simulink model "vkr_ch2_sync_custom"  (R2025b)
settings: Solver=FixedStepDiscrete  StartTime=0.0  StopTime=Nsym/Rs  FixedStep=1/Fs_tx  RelTol=1e-3
values from neighbouring files (symbols this model uses):
  Fs_tx = Rs * sps_tx    (= 8000000)    [params_tx.m]    (also in test_sync_loop.m)
  k_bits = log2(M)    [compare_all_architectures.m]    (also in compare_round_period_ber.m; compare_sync_direct.m; params_tx.m; run_ber_curve.m)
  Nsym = 10000    [params_tx.m]    (also in run_dynamics.m = 2000; run_sco_test.m = 30000; test_modelsim_io.m = 5000; test_rice_loop.m = 5000)
  rolloff = 0.35    [compare_all_architectures.m]    (also in compare_round_period_ber.m; compare_sync_direct.m; params_tx.m; process_real_data.m = 0.2)
  Rs = 1e6    (= 1000000)    [params_tx.m]    (also in test_sync_loop.m)
  sps_tx = 40    [compare_all_architectures.m]    (also in compare_round_period_ber.m; compare_sync_direct.m = 8; params_tx.m = 8; run_ber_curve.m = 8)
  timing_offset = 0.3    [compare_all_architectures.m]    (also in compare_round_period_ber.m; compare_sync_direct.m; params_tx.m; run_ber_curve.m)
libraries: commfilt2 x2, commchan3 x1, commrandsrc3 x1, commdigbbndpm3 x1, commsync2 x1, dspsigops x1
settings Model: Creator=Gostie2k  LastModifiedBy=t-kudimov

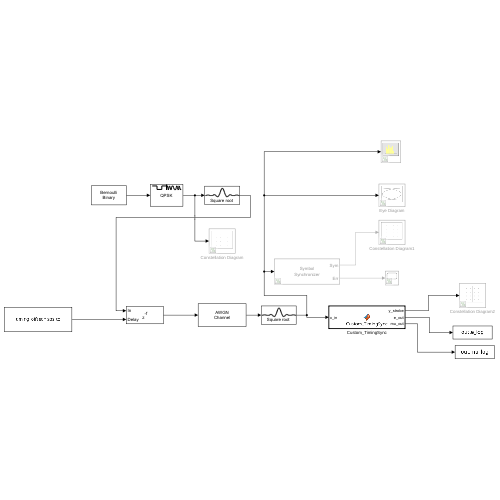
[thumbnail: Simulink's stored preview of the top-level diagram]
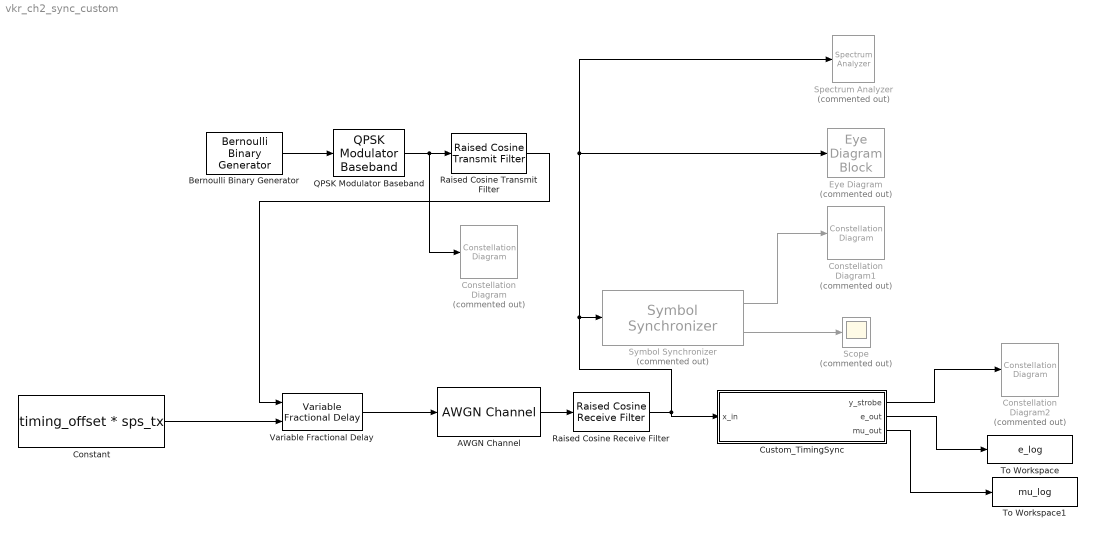
== system vkr_ch2_sync_custom ==
  AWGN Channel : commchan3/AWGN Channel  LegacyMode=off  NoiseMethod="Signal to noise ratio  (Eb/No)"  noiseMode="Signal to noise ratio  (SNR)"  EbNo=EbNo_dB  EsNo=10  SNR=10  BitsPerSymbol=k_bits  SignalPower=1  SpecifySymbolPeriod=off  SamplesPerSymbol=sps_tx  SymbolPeriod=1  VarianceSource=Parameter  Variance=1  RandomStream=Global stream  Seed=67  SimulateUsing=Code generation
  Bernoulli Binary Generator : commrandsrc3/Bernoulli Binary Generator  ProbabilityOfZero=0.5  SeedSource=Parameter  Seed=12345  SampleTime=1/(Rs*k_bits)  SamplesPerFrame=k_bits*Nsym  OutputDataType=double  SimulateUsing=Interpreted execution
  Constant : Constant  Value=timing_offset * sps_tx  OutDataTypeStr=double  SampleTime=1/Fs_tx
  Constellation Diagram : ConstellationDiagram  Commented=on  WindowPosition=[481.000000,476.000000,600.000000,605.000000,]  ScopeFrameLocation=window  ShowLegend=on
  Constellation Diagram1 : ConstellationDiagram  Commented=on  WindowPosition=[74.000000,-92.000000,600.000000,605.000000,]  ScopeFrameLocation=window  ShowLegend=on
  Constellation Diagram2 : ConstellationDiagram  Commented=on  WindowPosition=[1620.000000,-218.000000,600.000000,605.000000,]  ScopeFrameLocation=window  ShowLegend=on
  Custom_TimingSync : MATLAB Function  TreatAsAtomicUnit=on
  Eye Diagram : EyeDiagramBlock  Commented=on  WindowPosition=[1081.000000,-530.000000,1920.000000,1011.000000,]  ScopeFrameLocation=window  SamplesPerSymbol=2  TracesToDisplay=200  ColorFading=on
  QPSK Modulator Baseband : commdigbbndpm3/QPSK Modulator Baseband  InType=Bit  Enc=Gray  Ph=pi/4  outDtype=double  outWordLen=16  outUDDataType=sfix(16)  outFracLenMode=Best precision  outFracLen=15  outDataTypeStr=double  outLastDataTypeStr=double
  Raised Cosine Receive Filter : commfilt2/Raised Cosine Receive Filter  filtType=Square root  R=rolloff  filtSpan=span  N=sps_tx  downFactor=decim  downOffset=0  filterGain=1/sqrt(sps_tx)  InputProcessing=Columns as channels (frame based)  RateOptions=Allow multirate processing  framing=Mute  checkCoeff=off  variableName=rcRxFilt  currentFiltSpan=10  D=5  inputOffset=0  sampMode=Mute  saveAsFlag=0  rateMode=Downsampling  checkGain=Normalized  launchFVT=on  roundingMode=Floor  overflowMode=off  coeffDataTypeStr=Inherit: Same word length as input  coeffMin=[]  coeffMax=[]  coeffLastDataTypeStr=Inherit: Same word length as input  accumDataTypeStr=Inherit: Same as product output  accumLastDataTypeStr=Inherit: Same as product output  outputDataTypeStr=Inherit: Same as accumulator  outputMin=[]  outputMax=[]  outputLastDataTypeStr=Inherit: Same as accumulator
  Raised Cosine Transmit Filter : commfilt2/Raised Cosine Transmit Filter  filtType=Square root  R=rolloff  filtSpan=span  N=sps_tx  filterGain=sqrt(sps_tx)  InputProcessing=Columns as channels (frame based)  RateOptions=Enforce single-rate processing  framing=Mute  checkCoeff=off  variableName=rcTxFilt  checkGain=Normalized  sampMode=Mute  saveAsFlag=0  currentFiltSpan=10  D=(10)/2  launchFVT=on  roundingMode=Floor  overflowMode=off  coeffDataTypeStr=Inherit: Same word length as input  coeffMin=[]  coeffMax=[]  coeffLastDataTypeStr=Inherit: Same word length as input  outputDataTypeStr=Inherit: Same as accumulator  outputMin=[]  outputMax=[]  outputLastDataTypeStr=Inherit: Same as accumulator
  Scope : Scope  Commented=on
  Spectrum Analyzer : SpectrumAnalyzer  Commented=on  WindowPosition=[1081.000000,-530.000000,1920.000000,1011.000000,]  ScopeFrameLocation=window  SampleRateSource=Property  SampleRate=Fs_tx  WindowInvariantSamplesPerUpdate=on  Span=8000000  StartFrequency=-4000000  StopFrequency=4000000  MaximizeAxes=On  YLimits=[-95.1141 18.0217]
  Symbol Synchronizer : commsync2/Symbol Synchronizer  Commented=on  Modulation=PAM/PSK/QAM  TimingErrorDetector=Gardner (non-data-aided)  SamplesPerSymbol=sps_rx  DampingFactor=zeta  NormalizedLoopBandwidth=BnT  DetectorGain=2.7  TimingErrorOutputPort=on  SimulateUsing=Code generation
  To Workspace : ToWorkspace  VariableName=e_log  SampleTime=-1
  To Workspace1 : ToWorkspace  VariableName=mu_log  SampleTime=-1
  Variable Fractional Delay : dspsigops/Variable Fractional Delay  mode=OBSOLETE  modeActive=FIR  L=4  FarrowL=4  R=10  alpha=1  dmax=32  InputProcessing=Columns as channels (frame based)  ic=0  noDFT=off  fallbackFIR=Clip to the minimum value necessary for centered kernel  fallbackFarrow=Clip to the minimum value necessary for centered kernel  roundingMode=Zero  overflowMode=off
  wires:
  Variable Fractional Delay/1 -> AWGN Channel/1
  Bernoulli Binary Generator/1 -> QPSK Modulator Baseband/1
  QPSK Modulator Baseband/1 -> Constellation Diagram/1, Raised Cosine Transmit Filter/1
  Constant/1 -> Variable Fractional Delay/2
  AWGN Channel/1 -> Raised Cosine Receive Filter/1
  Raised Cosine Transmit Filter/1 -> Variable Fractional Delay/1
  Raised Cosine Receive Filter/1 -> Custom_TimingSync/1(x_in), Spectrum Analyzer/1, Eye Diagram/1, Symbol Synchronizer/1
  Symbol Synchronizer/2 -> Scope/1
  Symbol Synchronizer/1 -> Constellation Diagram1/1
  Custom_TimingSync/1(y_strobe) -> Constellation Diagram2/1
  Custom_TimingSync/2(e_out) -> To Workspace/1
  Custom_TimingSync/3(mu_out) -> To Workspace1/1

== matlab function vkr_ch2_sync_custom/Custom_TimingSync ==
  data: x_in input; y_strobe output; e_out output; mu_out output
function [y_strobe, e_out, mu_out] = Custom_TimingSync(x_in)
%#codegen
% =====================================================================
% Custom Timing Synchronizer — собственная реализация петли Gardner
% Заход 2: Farrow + NCO + Gardner TED, петля РАЗОМКНУТА (PI выключен)
%
% Вход:  x_in     — вектор комплексных отсчётов с RRC Rx (frame-based, 2 sps)
% Выходы:
%   y_strobe — стробированные символы (один отсчёт на символ, остальные нули)
%   e_out    — сигнал ошибки Gardner TED (для наблюдения)
%   mu_out   — текущее значение mu (для наблюдения)
% =====================================================================

%% Persistent: линия задержки интерполятора Фарроу
persistent x_n x_nm1 x_nm2 x_nm3

%% Persistent: состояние NCO
persistent eta            % регистр счётчика NCO (от 0 до 1)
persistent mu             % текущее значение дробной задержки
persistent strobe_flag    % флаг "сейчас strobe-такт" (true = решающий, false = промежуточный)

%% Persistent: история интерполированных отсчётов для Gardner TED
persistent y_strobe_curr  % текущий "решающий" отсчёт (на стробе)
persistent y_strobe_prev  % предыдущий "решающий" отсчёт
persistent y_mid          % промежуточный отсчёт (между стробами)

%% Инициализация при первом вызове
if isempty(x_n)
    x_n   = complex(0, 0);
    x_nm1 = complex(0, 0);
    x_nm2 = complex(0, 0);
    x_nm3 = complex(0, 0);
    eta          = 1.0;          % стартуем с полного регистра
    mu           = 0.0;
    strobe_flag  = false;        % первый отсчёт будет промежуточным
    y_strobe_curr = complex(0, 0);
    y_strobe_prev = complex(0, 0);
    y_mid         = complex(0, 0);
end

%% Параметры (на этом заходе W фиксированный, петля разомкнута)
sps   = 2;                       % отсчётов на символ
W     = 1/sps;                   % фиксированный шаг NCO (= 0.5)

%% Подготовка выходных векторов
N = length(x_in);
y_strobe = complex(zeros(N, 1));
e_out    = zeros(N, 1);
mu_out   = zeros(N, 1);

%% Главный цикл по отсчётам кадра
for n = 1:N
    
    % === 1. Сдвиг линии задержки и новый вход ===
    x_nm3 = x_nm2;
    x_nm2 = x_nm1;
    x_nm1 = x_n;
    x_n   = x_in(n);
    
    % === 2. Кубический Farrow с текущим mu ===
    v3 =  (1/6)*x_n - (1/2)*x_nm1 + (1/2)*x_nm2 - (1/6)*x_nm3;
    v2 =          0 + (1/2)*x_nm1 -        x_nm2 + (1/2)*x_nm3;
    v1 = -(1/6)*x_n +        x_nm1 - (1/2)*x_nm2 - (1/3)*x_nm3;
    v0 =                                   x_nm2;
    
    y_interp = ((v3*mu + v2)*mu + v1)*mu + v0;
    
    % === 3. NCO: декремент регистра ===
    eta_old = eta;
    eta_new = eta - W;
    
    % === 4. Проверка underflow ===
    if eta_new < 0
        % underflow: формируется новый strobe-момент
        mu = eta_old / W;        % дробная задержка для следующего интерполяции
        eta = eta_new + 1.0;     % восстановление в положительный диапазон (mod 1)
        
        % Переключение фазы: каждый второй underflow - "решающий" strobe
        strobe_flag = ~strobe_flag;
        
        if strobe_flag
            % Это "решающий" strobe-отсчёт: текущий y_interp = центр символа
            y_strobe_prev = y_strobe_curr;
            y_strobe_curr = y_interp;
            y_strobe(n)   = y_interp;     % выдаём на выход
            
            % === 5. Gardner TED: вычисление ошибки ===
            % e(k) = Re{ y_mid * conj(y_strobe_curr - y_strobe_prev) }
            e_out(n) = real(y_mid * conj(y_strobe_curr - y_strobe_prev));
        else
            % Это "промежуточный" отсчёт: запоминаем для следующего вычисления e(k)
            y_mid = y_interp;
        end
    else
        % Нет underflow: просто продвигаем eta
        eta = eta_new;
    end
    
    mu_out(n) = mu;
    
end

end
